simulink model "untitled"  (R2020b)
settings: Solver=VariableStepAuto  StartTime=0.0  StopTime=10.0  RelTol=1e-3
libraries: visionsources x1
settings Model: Creator=anne  LastModifiedBy=anne

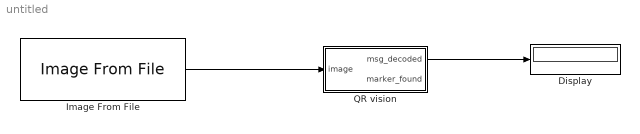
== system untitled ==
  Display : Display
  Image From File : visionsources/Image From File  Tag=vipblks_nd  FileName=/home/anne/Documents/uni/2.kan/GNC/project/Landmark_navigation_vison/jpg.png  Ts=inf  imagePorts=One multidimensional signal  OutPortLabels=R|G|B  ImageDataType=Inherit from input image  sdImageDataType=uint(8)  Signed=on  WordLength=16  FractionLengthMode=User-defined  FractionLength=15
  QR vision : Subsystem
  wires:
  Image From File/1 -> QR vision/1(image)
  QR vision/1(msg_decoded) -> Display/1

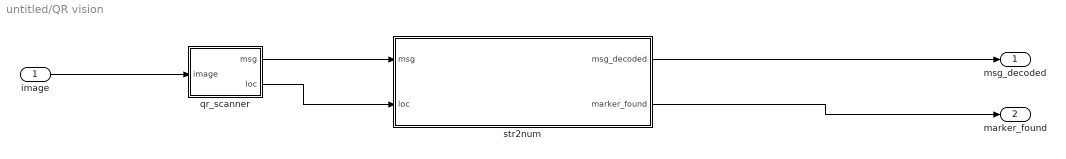
== system untitled/QR vision ==
  image : Inport
  qr_scanner : MATLAB Function  TreatAsAtomicUnit=on
  str2num : MATLAB Function  TreatAsAtomicUnit=on
  msg_decoded : Outport
  marker_found : Outport  Port=2
  wires:
  qr_scanner/1(msg) -> str2num/1(msg)
  image/1 -> qr_scanner/1(image)
  str2num/1(msg_decoded) -> msg_decoded/1
  str2num/2(marker_found) -> marker_found/1
  qr_scanner/2(loc) -> str2num/2(loc)

== matlab function untitled/QR vision/qr_scanner ==
  data: image input; msg output; loc output
function [msg, loc] = fcn(image)
%%image = imreader(image_ra)
[rows, cols] = size(image);

roi = [1,1,cols, rows];
[msg,~,loc] = readBarcode(image, roi,"QR-CODE"); 
end

== matlab function untitled/QR vision/str2num ==
  data: msg input; msg_decoded output; loc input; marker_found output
function [msg_decoded, marker_found] = fcn(msg,loc)
    msg_decoded = [];
    if(size(msg) == 0)
        marker_found = -1;
    else
        raw_msg = split(msg,",");
        marker_found = 1;
        [size_r,si] = size(raw_msg)
        for i = 1:size_r
            msg_decoded = [msg_decoded str2num(raw_msg(i))];
        end
        
    end
       
end
